simulink library "Common_Library"  (Simulink 8.1)
settings: Solver=ode45  StartTime=0.0  StopTime=10.0  RelTol=1e-3
values from neighbouring files (symbols this model uses):
  address_0x00 = MOVcr    [ROM.m]
  address_0x01 = 10    [ROM.m]
  address_0x02 = REG_A    [ROM.m]
  address_0x03 = MOVcr    [ROM.m]
  address_0x04 = 3    [ROM.m]
  address_0x05 = REG_B    [ROM.m]
  address_0x06 = ADDcr    [ROM.m]
  address_0x07 = 50    [ROM.m]
  address_0x08 = REG_B    [ROM.m]
  address_0x09 = ADDrr    [ROM.m]
  address_0x0A = REG_A    [ROM.m]
  address_0x0B = REG_B    [ROM.m]
  address_0x0C = 0    [ROM.m]
  address_0x0D = 0    [ROM.m]
  address_0x0E = 0    [ROM.m]
  address_0x0F = 177    [ROM.m]
libraries: Common_Library x115, Computer_Library x85, commutil2 x67, simulink_extras x1
(part 2 of 3)

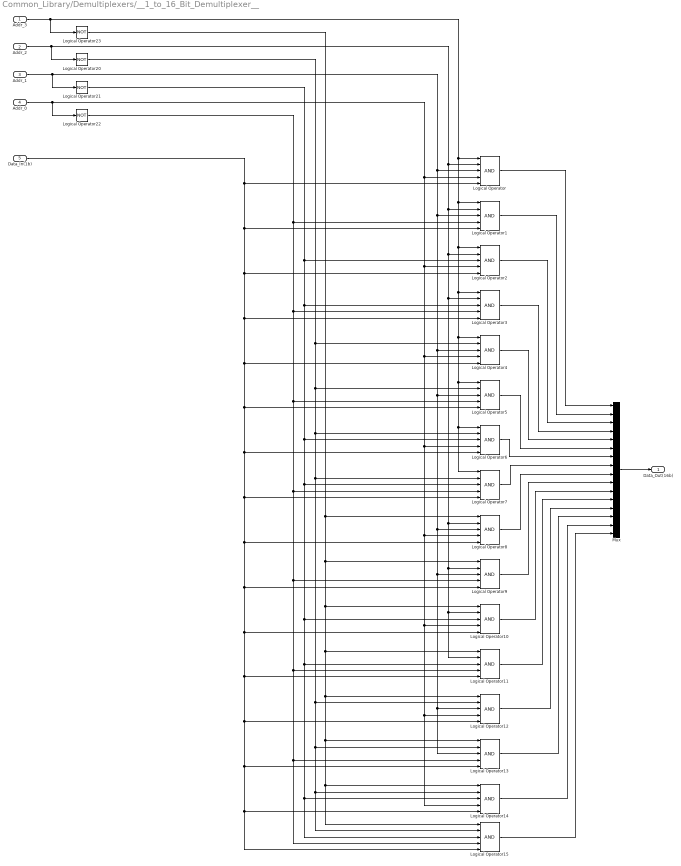
== system Common_Library/Demultiplexers/__1_to_16_Bit_Demultiplexer__ ==
  Addr_3 : Inport
  Addr_2 : Inport  Port=2
  Addr_1 : Inport  Port=3
  Addr_0 : Inport  Port=4
  Data_In(1b) : Inport  Port=5
  Logical Operator{,1..15} (16 alike) : Logic  Inputs=5  IconShape=distinctive  AllPortsSameDT=off  OutDataTypeStr=boolean
  Logical Operator{20..23} (4 alike) : Logic  Operator=NOT  Inputs=4  IconShape=distinctive  AllPortsSameDT=off  OutDataTypeStr=boolean
  Mux : Mux  Inputs=16
  Data_Out(16b) : Outport
  wires:
  Mux/1 -> Data_Out(16b)/1
  Logical Operator22/1 -> Logical Operator15/4, Logical Operator13/4, Logical Operator11/4, Logical Operator9/4, Logical Operator7/4, Logical Operator5/4, Logical Operator3/4, Logical Operator1/4
  Addr_0/1 -> Logical Operator14/4, Logical Operator12/4, Logical Operator10/4, Logical Operator8/4, Logical Operator6/4, Logical Operator4/4, Logical Operator2/4, Logical Operator/4, Logical Operator22/1
  Logical Operator21/1 -> Logical Operator15/3, Logical Operator14/3, Logical Operator11/3, Logical Operator10/3, Logical Operator7/3, Logical Operator6/3, Logical Operator3/3, Logical Operator2/3
  Addr_1/1 -> Logical Operator13/3, Logical Operator12/3, Logical Operator9/3, Logical Operator8/3, Logical Operator5/3, Logical Operator4/3, Logical Operator1/3, Logical Operator/3, Logical Operator21/1
  Logical Operator20/1 -> Logical Operator15/2, Logical Operator14/2, Logical Operator13/2, Logical Operator12/2, Logical Operator7/2, Logical Operator6/2, Logical Operator5/2, Logical Operator4/2
  Addr_2/1 -> Logical Operator11/2, Logical Operator10/2, Logical Operator9/2, Logical Operator8/2, Logical Operator3/2, Logical Operator2/2, Logical Operator1/2, Logical Operator/2, Logical Operator20/1
  Logical Operator23/1 -> Logical Operator15/1, Logical Operator14/1, Logical Operator13/1, Logical Operator12/1, Logical Operator11/1, Logical Operator10/1, Logical Operator9/1, Logical Operator8/1
  Addr_3/1 -> Logical Operator7/1, Logical Operator6/1, Logical Operator5/1, Logical Operator4/1, Logical Operator3/1, Logical Operator2/1, Logical Operator1/1, Logical Operator/1, Logical Operator23/1
  Data_In(1b)/1 -> Logical Operator/5, Logical Operator3/5, Logical Operator7/5, Logical Operator8/5, Logical Operator9/5, Logical Operator10/5, Logical Operator11/5, Logical Operator15/5, Logical Operator14/5, Logical Operator13/5, Logical Operator12/5, Logical Operator6/5, Logical Operator5/5, Logical Operator4/5, Logical Operator2/5, Logical Operator1/5
  Logical Operator15/1 -> Mux/16
  Logical Operator14/1 -> Mux/15
  Logical Operator13/1 -> Mux/14
  Logical Operator/1 -> Mux/1
  Logical Operator1/1 -> Mux/2
  Logical Operator2/1 -> Mux/3
  Logical Operator3/1 -> Mux/4
  Logical Operator4/1 -> Mux/5
  Logical Operator12/1 -> Mux/13
  Logical Operator11/1 -> Mux/12
  Logical Operator5/1 -> Mux/6
  Logical Operator10/1 -> Mux/11
  Logical Operator9/1 -> Mux/10
  Logical Operator6/1 -> Mux/7
  Logical Operator8/1 -> Mux/9
  Logical Operator7/1 -> Mux/8

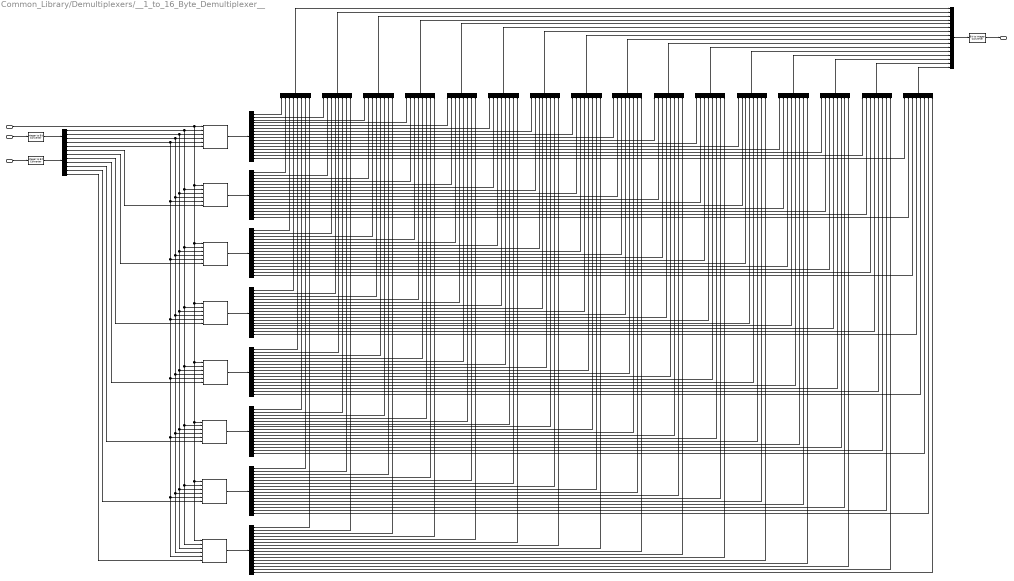
== system Common_Library/Demultiplexers/__1_to_16_Byte_Demultiplexer__ ==
  Enable : Inport
  Addr(4b) : Inport  Port=2
  Data_In(1B) : Inport  Port=3
  1_to_16_Bit_Demultiplexer(Bit_0) : Common_Library/Demultiplexers/1_to_16_Bit_Demultiplexer
  1_to_16_Bit_Demultiplexer(Bit_1) : Common_Library/Demultiplexers/1_to_16_Bit_Demultiplexer
  1_to_16_Bit_Demultiplexer(Bit_2) : Common_Library/Demultiplexers/1_to_16_Bit_Demultiplexer
  1_to_16_Bit_Demultiplexer(Bit_3) : Common_Library/Demultiplexers/1_to_16_Bit_Demultiplexer
  1_to_16_Bit_Demultiplexer(Bit_4) : Common_Library/Demultiplexers/1_to_16_Bit_Demultiplexer
  1_to_16_Bit_Demultiplexer(Bit_5) : Common_Library/Demultiplexers/1_to_16_Bit_Demultiplexer
  1_to_16_Bit_Demultiplexer(Bit_6) : Common_Library/Demultiplexers/1_to_16_Bit_Demultiplexer
  1_to_16_Bit_Demultiplexer(Bit_7) : Common_Library/Demultiplexers/1_to_16_Bit_Demultiplexer
  Bit to Integer Converter : commutil2/Bit to Integer Converter  nbits=8  bitOrder=MSB first  signedOutputValues=Unsigned  outDtype=uint8  outDtypeSigned=Inherit via internal rule
  Bit_{0..7} (8 alike) : Demux  Outputs=16
  Byte_{0..15} (16 alike) : Mux  Inputs=8
  Demux1 : Demux  Outputs=8
  Demux17 : Demux
  Integer to Bit Converter5 : commutil2/Integer to Bit Converter  nbits=4  signedInputValues=Unsigned  bitOrder=MSB first  outDtype=int8
  Integer to Bit Converter7 : commutil2/Integer to Bit Converter  nbits=8  signedInputValues=Unsigned  bitOrder=MSB first  outDtype=boolean
  Mux1 : Mux  Inputs=16
  Data_Out(16B) : Outport
  wires:
  Bit to Integer Converter/1 -> Data_Out(16B)/1
  Mux1/1 -> Bit to Integer Converter/1
  Addr(4b)/1 -> Integer to Bit Converter5/1
  Integer to Bit Converter5/1 -> Demux17/1
  Enable/1 -> 1_to_16_Bit_Demultiplexer(Bit_0)/1, 1_to_16_Bit_Demultiplexer(Bit_1)/1, 1_to_16_Bit_Demultiplexer(Bit_2)/1, 1_to_16_Bit_Demultiplexer(Bit_3)/1, 1_to_16_Bit_Demultiplexer(Bit_4)/1, 1_to_16_Bit_Demultiplexer(Bit_5)/1, 1_to_16_Bit_Demultiplexer(Bit_6)/1, 1_to_16_Bit_Demultiplexer(Bit_7)/1
  Demux1/4 -> 1_to_16_Bit_Demultiplexer(Bit_4)/6
  Demux1/5 -> 1_to_16_Bit_Demultiplexer(Bit_3)/6
  Demux1/6 -> 1_to_16_Bit_Demultiplexer(Bit_2)/6
  Demux1/7 -> 1_to_16_Bit_Demultiplexer(Bit_1)/6
  Demux1/8 -> 1_to_16_Bit_Demultiplexer(Bit_0)/6
  Demux1/3 -> 1_to_16_Bit_Demultiplexer(Bit_5)/6
  Demux1/2 -> 1_to_16_Bit_Demultiplexer(Bit_6)/6
  Demux1/1 -> 1_to_16_Bit_Demultiplexer(Bit_7)/6
  Byte_15/1 -> Mux1/1
  Byte_14/1 -> Mux1/2
  Byte_13/1 -> Mux1/3
  Byte_12/1 -> Mux1/4
  Byte_11/1 -> Mux1/5
  Byte_10/1 -> Mux1/6
  Byte_9/1 -> Mux1/7
  Byte_8/1 -> Mux1/8
  Byte_7/1 -> Mux1/9
  Byte_6/1 -> Mux1/10
  Byte_5/1 -> Mux1/11
  Byte_4/1 -> Mux1/12
  Byte_3/1 -> Mux1/13
  Byte_2/1 -> Mux1/14
  Byte_1/1 -> Mux1/15
  Byte_0/1 -> Mux1/16
  Bit_0/16 -> Byte_0/8
  Bit_0/15 -> Byte_1/8
  Bit_0/14 -> Byte_2/8
  Bit_0/13 -> Byte_3/8
  Bit_0/12 -> Byte_4/8
  Bit_0/11 -> Byte_5/8
  Bit_0/10 -> Byte_6/8
  Bit_0/9 -> Byte_7/8
  Bit_0/8 -> Byte_8/8
  Bit_0/7 -> Byte_9/8
  Bit_0/6 -> Byte_10/8
  Bit_0/5 -> Byte_11/8
  Bit_0/4 -> Byte_12/8
  Bit_0/3 -> Byte_13/8
  Bit_0/2 -> Byte_14/8
  Bit_0/1 -> Byte_15/8
  Bit_1/16 -> Byte_0/7
  Bit_1/15 -> Byte_1/7
  Bit_1/14 -> Byte_2/7
  Bit_1/13 -> Byte_3/7
  Bit_1/12 -> Byte_4/7
  Bit_1/11 -> Byte_5/7
  Bit_1/10 -> Byte_6/7
  Bit_1/9 -> Byte_7/7
  Bit_1/8 -> Byte_8/7
  Bit_1/7 -> Byte_9/7
  Bit_1/6 -> Byte_10/7
  Bit_1/5 -> Byte_11/7
  Bit_1/4 -> Byte_12/7
  Bit_1/3 -> Byte_13/7
  Bit_1/2 -> Byte_14/7
  Bit_1/1 -> Byte_15/7
  Bit_2/16 -> Byte_0/6
  Bit_2/15 -> Byte_1/6
  Bit_2/14 -> Byte_2/6
  Bit_2/13 -> Byte_3/6
  Bit_2/12 -> Byte_4/6
  Bit_2/11 -> Byte_5/6
  Bit_2/10 -> Byte_6/6
  Bit_2/9 -> Byte_7/6
  Bit_2/8 -> Byte_8/6
  Bit_2/7 -> Byte_9/6
  Bit_2/6 -> Byte_10/6
  Bit_2/5 -> Byte_11/6
  Bit_2/4 -> Byte_12/6
  Bit_2/3 -> Byte_13/6
  Bit_2/2 -> Byte_14/6
  Bit_2/1 -> Byte_15/6
  Bit_3/16 -> Byte_0/5
  Bit_3/15 -> Byte_1/5
  Bit_3/14 -> Byte_2/5
  Bit_3/13 -> Byte_3/5
  Bit_3/12 -> Byte_4/5
  Bit_3/11 -> Byte_5/5
  Bit_3/10 -> Byte_6/5
  Bit_3/9 -> Byte_7/5
  Bit_3/8 -> Byte_8/5
  Bit_3/7 -> Byte_9/5
  Bit_3/6 -> Byte_10/5
  Bit_3/5 -> Byte_11/5
  Bit_3/4 -> Byte_12/5
  Bit_3/3 -> Byte_13/5
  Bit_3/2 -> Byte_14/5
  Bit_3/1 -> Byte_15/5
  Bit_4/16 -> Byte_0/4
  Bit_4/15 -> Byte_1/4
  Bit_4/14 -> Byte_2/4
  Bit_4/13 -> Byte_3/4
  Bit_4/12 -> Byte_4/4
  Bit_4/11 -> Byte_5/4
  Bit_4/10 -> Byte_6/4
  Bit_4/9 -> Byte_7/4
  Bit_4/8 -> Byte_8/4
  Bit_4/7 -> Byte_9/4
  Bit_4/6 -> Byte_10/4
  Bit_4/5 -> Byte_11/4
  Bit_4/4 -> Byte_12/4
  Bit_4/3 -> Byte_13/4
  Bit_4/2 -> Byte_14/4
  Bit_4/1 -> Byte_15/4
  Bit_5/16 -> Byte_0/3
  Bit_5/15 -> Byte_1/3
  Bit_5/14 -> Byte_2/3
  Bit_5/13 -> Byte_3/3
  Bit_5/12 -> Byte_4/3
  Bit_5/11 -> Byte_5/3
  Bit_5/10 -> Byte_6/3
  Bit_5/9 -> Byte_7/3
  Bit_5/8 -> Byte_8/3
  Bit_5/7 -> Byte_9/3
  Bit_5/6 -> Byte_10/3
  Bit_5/5 -> Byte_11/3
  Bit_5/4 -> Byte_12/3
  Bit_5/3 -> Byte_13/3
  Bit_5/2 -> Byte_14/3
  Bit_5/1 -> Byte_15/3
  Bit_6/16 -> Byte_0/2
  Bit_6/15 -> Byte_1/2
  Bit_6/14 -> Byte_2/2
  Bit_6/13 -> Byte_3/2
  Bit_6/12 -> Byte_4/2
  Bit_6/11 -> Byte_5/2
  Bit_6/10 -> Byte_6/2
  Bit_6/9 -> Byte_7/2
  Bit_6/8 -> Byte_8/2
  Bit_6/7 -> Byte_9/2
  Bit_6/6 -> Byte_10/2
  Bit_6/5 -> Byte_11/2
  Bit_6/4 -> Byte_12/2
  Bit_6/3 -> Byte_13/2
  Bit_6/2 -> Byte_14/2
  Bit_6/1 -> Byte_15/2
  Bit_7/16 -> Byte_0/1
  Bit_7/15 -> Byte_1/1
  Bit_7/14 -> Byte_2/1
  Bit_7/13 -> Byte_3/1
  Bit_7/12 -> Byte_4/1
  Bit_7/11 -> Byte_5/1
  Bit_7/10 -> Byte_6/1
  Bit_7/9 -> Byte_7/1
  Bit_7/8 -> Byte_8/1
  Bit_7/7 -> Byte_9/1
  Bit_7/6 -> Byte_10/1
  Bit_7/5 -> Byte_11/1
  Bit_7/4 -> Byte_12/1
  Bit_7/3 -> Byte_13/1
  Bit_7/2 -> Byte_14/1
  Bit_7/1 -> Byte_15/1
  1_to_16_Bit_Demultiplexer(Bit_0)/1 -> Bit_0/1
  1_to_16_Bit_Demultiplexer(Bit_1)/1 -> Bit_1/1
  1_to_16_Bit_Demultiplexer(Bit_2)/1 -> Bit_2/1
  1_to_16_Bit_Demultiplexer(Bit_3)/1 -> Bit_3/1
  1_to_16_Bit_Demultiplexer(Bit_4)/1 -> Bit_4/1
  1_to_16_Bit_Demultiplexer(Bit_5)/1 -> Bit_5/1
  1_to_16_Bit_Demultiplexer(Bit_6)/1 -> Bit_6/1
  1_to_16_Bit_Demultiplexer(Bit_7)/1 -> Bit_7/1
  Integer to Bit Converter7/1 -> Demux1/1
  Data_In(1B)/1 -> Integer to Bit Converter7/1
  Demux17/4 -> 1_to_16_Bit_Demultiplexer(Bit_7)/5, 1_to_16_Bit_Demultiplexer(Bit_0)/5, 1_to_16_Bit_Demultiplexer(Bit_1)/5, 1_to_16_Bit_Demultiplexer(Bit_2)/5, 1_to_16_Bit_Demultiplexer(Bit_3)/5, 1_to_16_Bit_Demultiplexer(Bit_4)/5, 1_to_16_Bit_Demultiplexer(Bit_5)/5, 1_to_16_Bit_Demultiplexer(Bit_6)/5
  Demux17/3 -> 1_to_16_Bit_Demultiplexer(Bit_7)/4, 1_to_16_Bit_Demultiplexer(Bit_0)/4, 1_to_16_Bit_Demultiplexer(Bit_1)/4, 1_to_16_Bit_Demultiplexer(Bit_2)/4, 1_to_16_Bit_Demultiplexer(Bit_3)/4, 1_to_16_Bit_Demultiplexer(Bit_4)/4, 1_to_16_Bit_Demultiplexer(Bit_5)/4, 1_to_16_Bit_Demultiplexer(Bit_6)/4
  Demux17/2 -> 1_to_16_Bit_Demultiplexer(Bit_7)/3, 1_to_16_Bit_Demultiplexer(Bit_1)/3, 1_to_16_Bit_Demultiplexer(Bit_0)/3, 1_to_16_Bit_Demultiplexer(Bit_2)/3, 1_to_16_Bit_Demultiplexer(Bit_3)/3, 1_to_16_Bit_Demultiplexer(Bit_4)/3, 1_to_16_Bit_Demultiplexer(Bit_5)/3, 1_to_16_Bit_Demultiplexer(Bit_6)/3
  Demux17/1 -> 1_to_16_Bit_Demultiplexer(Bit_7)/2, 1_to_16_Bit_Demultiplexer(Bit_0)/2, 1_to_16_Bit_Demultiplexer(Bit_1)/2, 1_to_16_Bit_Demultiplexer(Bit_2)/2, 1_to_16_Bit_Demultiplexer(Bit_3)/2, 1_to_16_Bit_Demultiplexer(Bit_4)/2, 1_to_16_Bit_Demultiplexer(Bit_5)/2, 1_to_16_Bit_Demultiplexer(Bit_6)/2

== system Common_Library/Demultiplexers/__1_to_256_Bit_Demultiplexer__ ==
  Address(8b) : Inport
  Data_In(1b) : Inport  Port=2
  1_to_16_Bit_Demultiplexer{,1..16} (17 alike) : Computer_Library/Demultiplexers/1_to_16_Bit_Demultiplexer
  Constant : Constant
  Demux1 : Demux  Outputs=16
  Demux17 : Demux  Outputs=8
  Mux : Mux  Inputs=16
  Data_Out(256b) : Outport  OutDataTypeStr=boolean
  wires:
  Mux/1 -> Data_Out(256b)/1
  Constant/1 -> 1_to_16_Bit_Demultiplexer16/1
  Demux17/4 -> 1_to_16_Bit_Demultiplexer16/5
  Demux17/3 -> 1_to_16_Bit_Demultiplexer16/4
  Demux17/2 -> 1_to_16_Bit_Demultiplexer16/3
  Demux17/1 -> 1_to_16_Bit_Demultiplexer16/2
  Demux1/16 -> 1_to_16_Bit_Demultiplexer15/1
  Demux1/15 -> 1_to_16_Bit_Demultiplexer14/1
  Demux1/14 -> 1_to_16_Bit_Demultiplexer13/1
  Demux1/13 -> 1_to_16_Bit_Demultiplexer12/1
  Demux1/12 -> 1_to_16_Bit_Demultiplexer11/1
  Demux1/11 -> 1_to_16_Bit_Demultiplexer10/1
  Demux1/10 -> 1_to_16_Bit_Demultiplexer9/1
  Demux1/9 -> 1_to_16_Bit_Demultiplexer8/1
  Demux1/8 -> 1_to_16_Bit_Demultiplexer7/1
  Demux1/7 -> 1_to_16_Bit_Demultiplexer6/1
  Demux1/6 -> 1_to_16_Bit_Demultiplexer5/1
  Demux1/5 -> 1_to_16_Bit_Demultiplexer4/1
  Demux1/4 -> 1_to_16_Bit_Demultiplexer3/1
  Demux1/3 -> 1_to_16_Bit_Demultiplexer2/1
  Demux1/2 -> 1_to_16_Bit_Demultiplexer1/1
  Demux1/1 -> 1_to_16_Bit_Demultiplexer/1
  1_to_16_Bit_Demultiplexer16/1 -> Demux1/1
  Data_In(1b)/1 -> 1_to_16_Bit_Demultiplexer16/6, 1_to_16_Bit_Demultiplexer/6, 1_to_16_Bit_Demultiplexer2/6, 1_to_16_Bit_Demultiplexer3/6, 1_to_16_Bit_Demultiplexer4/6, 1_to_16_Bit_Demultiplexer5/6, 1_to_16_Bit_Demultiplexer6/6, 1_to_16_Bit_Demultiplexer7/6, 1_to_16_Bit_Demultiplexer8/6, 1_to_16_Bit_Demultiplexer9/6, 1_to_16_Bit_Demultiplexer10/6, 1_to_16_Bit_Demultiplexer11/6, 1_to_16_Bit_Demultiplexer12/6, 1_to_16_Bit_Demultiplexer13/6, 1_to_16_Bit_Demultiplexer14/6, 1_to_16_Bit_Demultiplexer15/6, 1_to_16_Bit_Demultiplexer1/6
  1_to_16_Bit_Demultiplexer/1 -> Mux/1
  1_to_16_Bit_Demultiplexer1/1 -> Mux/2
  1_to_16_Bit_Demultiplexer2/1 -> Mux/3
  1_to_16_Bit_Demultiplexer3/1 -> Mux/4
  1_to_16_Bit_Demultiplexer15/1 -> Mux/16
  1_to_16_Bit_Demultiplexer14/1 -> Mux/15
  1_to_16_Bit_Demultiplexer13/1 -> Mux/14
  1_to_16_Bit_Demultiplexer12/1 -> Mux/13
  1_to_16_Bit_Demultiplexer11/1 -> Mux/12
  1_to_16_Bit_Demultiplexer10/1 -> Mux/11
  1_to_16_Bit_Demultiplexer9/1 -> Mux/10
  1_to_16_Bit_Demultiplexer8/1 -> Mux/9
  1_to_16_Bit_Demultiplexer7/1 -> Mux/8
  1_to_16_Bit_Demultiplexer6/1 -> Mux/7
  1_to_16_Bit_Demultiplexer5/1 -> Mux/6
  1_to_16_Bit_Demultiplexer4/1 -> Mux/5
  Demux17/5 -> 1_to_16_Bit_Demultiplexer/2, 1_to_16_Bit_Demultiplexer7/2, 1_to_16_Bit_Demultiplexer9/2, 1_to_16_Bit_Demultiplexer10/2, 1_to_16_Bit_Demultiplexer14/2, 1_to_16_Bit_Demultiplexer15/2, 1_to_16_Bit_Demultiplexer13/2, 1_to_16_Bit_Demultiplexer12/2, 1_to_16_Bit_Demultiplexer11/2, 1_to_16_Bit_Demultiplexer8/2, 1_to_16_Bit_Demultiplexer6/2, 1_to_16_Bit_Demultiplexer5/2, 1_to_16_Bit_Demultiplexer4/2, 1_to_16_Bit_Demultiplexer3/2, 1_to_16_Bit_Demultiplexer2/2, 1_to_16_Bit_Demultiplexer1/2
  Demux17/6 -> 1_to_16_Bit_Demultiplexer/3, 1_to_16_Bit_Demultiplexer3/3, 1_to_16_Bit_Demultiplexer4/3, 1_to_16_Bit_Demultiplexer7/3, 1_to_16_Bit_Demultiplexer8/3, 1_to_16_Bit_Demultiplexer9/3, 1_to_16_Bit_Demultiplexer10/3, 1_to_16_Bit_Demultiplexer12/3, 1_to_16_Bit_Demultiplexer14/3, 1_to_16_Bit_Demultiplexer15/3, 1_to_16_Bit_Demultiplexer13/3, 1_to_16_Bit_Demultiplexer11/3, 1_to_16_Bit_Demultiplexer6/3, 1_to_16_Bit_Demultiplexer5/3, 1_to_16_Bit_Demultiplexer2/3, 1_to_16_Bit_Demultiplexer1/3
  Demux17/7 -> 1_to_16_Bit_Demultiplexer/4, 1_to_16_Bit_Demultiplexer2/4, 1_to_16_Bit_Demultiplexer3/4, 1_to_16_Bit_Demultiplexer4/4, 1_to_16_Bit_Demultiplexer7/4, 1_to_16_Bit_Demultiplexer8/4, 1_to_16_Bit_Demultiplexer9/4, 1_to_16_Bit_Demultiplexer10/4, 1_to_16_Bit_Demultiplexer12/4, 1_to_16_Bit_Demultiplexer14/4, 1_to_16_Bit_Demultiplexer15/4, 1_to_16_Bit_Demultiplexer13/4, 1_to_16_Bit_Demultiplexer11/4, 1_to_16_Bit_Demultiplexer6/4, 1_to_16_Bit_Demultiplexer5/4, 1_to_16_Bit_Demultiplexer1/4
  Demux17/8 -> 1_to_16_Bit_Demultiplexer/5, 1_to_16_Bit_Demultiplexer1/5, 1_to_16_Bit_Demultiplexer2/5, 1_to_16_Bit_Demultiplexer3/5, 1_to_16_Bit_Demultiplexer4/5, 1_to_16_Bit_Demultiplexer5/5, 1_to_16_Bit_Demultiplexer7/5, 1_to_16_Bit_Demultiplexer8/5, 1_to_16_Bit_Demultiplexer9/5, 1_to_16_Bit_Demultiplexer10/5, 1_to_16_Bit_Demultiplexer12/5, 1_to_16_Bit_Demultiplexer14/5, 1_to_16_Bit_Demultiplexer15/5, 1_to_16_Bit_Demultiplexer13/5, 1_to_16_Bit_Demultiplexer11/5, 1_to_16_Bit_Demultiplexer6/5
  Address(8b)/1 -> Demux17/1

== system Common_Library/Demultiplexers/__1_to_256_Byte_Demultiplexer__ ==
  Address(8b) : Inport
  Data_In(1B) : Inport  Port=2
  1_to_16_Bit_Demultiplexer16 : Computer_Library/Demultiplexers/1_to_16_Bit_Demultiplexer
  1_to_16_Byte_Demultiplexer{,1..15} (16 alike) : Computer_Library/Demultiplexers/1_to_16_Byte_Demultiplexer
  Bit to Integer Converter : commutil2/Bit to Integer Converter  nbits=4  bitOrder=MSB first  signedOutputValues=Unsigned  outDtype=uint8  outDtypeSigned=Inherit via internal rule
  Constant : Constant
  Demux1 : Demux  Outputs=16
  Demux17 : Demux  Outputs=8
  Integer to Bit Converter7 : commutil2/Integer to Bit Converter  nbits=8  signedInputValues=Unsigned  bitOrder=MSB first  outDtype=boolean
  Mux : Mux  Inputs=16
  Mux1 : Mux
  Data_Out(256B) : Outport  OutDataTypeStr=uint8
  wires:
  Mux1/1 -> Bit to Integer Converter/1
  Address(8b)/1 -> Integer to Bit Converter7/1
  Integer to Bit Converter7/1 -> Demux17/1
  Bit to Integer Converter/1 -> 1_to_16_Byte_Demultiplexer2/2, 1_to_16_Byte_Demultiplexer3/2, 1_to_16_Byte_Demultiplexer4/2, 1_to_16_Byte_Demultiplexer15/2, 1_to_16_Byte_Demultiplexer14/2, 1_to_16_Byte_Demultiplexer13/2, 1_to_16_Byte_Demultiplexer12/2, 1_to_16_Byte_Demultiplexer11/2, 1_to_16_Byte_Demultiplexer10/2, 1_to_16_Byte_Demultiplexer9/2, 1_to_16_Byte_Demultiplexer8/2, 1_to_16_Byte_Demultiplexer7/2, 1_to_16_Byte_Demultiplexer6/2, 1_to_16_Byte_Demultiplexer5/2, 1_to_16_Byte_Demultiplexer1/2, 1_to_16_Byte_Demultiplexer/2
  Demux17/8 -> Mux1/4
  Demux17/7 -> Mux1/3
  Demux17/6 -> Mux1/2
  Demux17/5 -> Mux1/1
  Demux17/3 -> 1_to_16_Bit_Demultiplexer16/4
  Demux17/4 -> 1_to_16_Bit_Demultiplexer16/5
  Demux17/2 -> 1_to_16_Bit_Demultiplexer16/3
  Demux17/1 -> 1_to_16_Bit_Demultiplexer16/2
  Mux/1 -> Data_Out(256B)/1
  Constant/1 -> 1_to_16_Bit_Demultiplexer16/6, 1_to_16_Bit_Demultiplexer16/1
  Demux1/16 -> 1_to_16_Byte_Demultiplexer15/1
  Demux1/15 -> 1_to_16_Byte_Demultiplexer14/1
  Demux1/14 -> 1_to_16_Byte_Demultiplexer13/1
  Demux1/13 -> 1_to_16_Byte_Demultiplexer12/1
  Demux1/12 -> 1_to_16_Byte_Demultiplexer11/1
  Demux1/11 -> 1_to_16_Byte_Demultiplexer10/1
  Demux1/10 -> 1_to_16_Byte_Demultiplexer9/1
  Demux1/9 -> 1_to_16_Byte_Demultiplexer8/1
  Demux1/8 -> 1_to_16_Byte_Demultiplexer7/1
  Demux1/7 -> 1_to_16_Byte_Demultiplexer6/1
  Demux1/6 -> 1_to_16_Byte_Demultiplexer5/1
  Demux1/5 -> 1_to_16_Byte_Demultiplexer4/1
  Demux1/4 -> 1_to_16_Byte_Demultiplexer3/1
  Demux1/3 -> 1_to_16_Byte_Demultiplexer2/1
  Demux1/2 -> 1_to_16_Byte_Demultiplexer1/1
  Demux1/1 -> 1_to_16_Byte_Demultiplexer/1
  1_to_16_Bit_Demultiplexer16/1 -> Demux1/1
  Data_In(1B)/1 -> 1_to_16_Byte_Demultiplexer/3, 1_to_16_Byte_Demultiplexer1/3, 1_to_16_Byte_Demultiplexer2/3, 1_to_16_Byte_Demultiplexer3/3, 1_to_16_Byte_Demultiplexer4/3, 1_to_16_Byte_Demultiplexer5/3, 1_to_16_Byte_Demultiplexer6/3, 1_to_16_Byte_Demultiplexer7/3, 1_to_16_Byte_Demultiplexer8/3, 1_to_16_Byte_Demultiplexer9/3, 1_to_16_Byte_Demultiplexer10/3, 1_to_16_Byte_Demultiplexer11/3, 1_to_16_Byte_Demultiplexer12/3, 1_to_16_Byte_Demultiplexer13/3, 1_to_16_Byte_Demultiplexer14/3, 1_to_16_Byte_Demultiplexer15/3
  1_to_16_Byte_Demultiplexer/1 -> Mux/1
  1_to_16_Byte_Demultiplexer1/1 -> Mux/2
  1_to_16_Byte_Demultiplexer2/1 -> Mux/3
  1_to_16_Byte_Demultiplexer3/1 -> Mux/4
  1_to_16_Byte_Demultiplexer15/1 -> Mux/16
  1_to_16_Byte_Demultiplexer14/1 -> Mux/15
  1_to_16_Byte_Demultiplexer13/1 -> Mux/14
  1_to_16_Byte_Demultiplexer12/1 -> Mux/13
  1_to_16_Byte_Demultiplexer11/1 -> Mux/12
  1_to_16_Byte_Demultiplexer10/1 -> Mux/11
  1_to_16_Byte_Demultiplexer9/1 -> Mux/10
  1_to_16_Byte_Demultiplexer8/1 -> Mux/9
  1_to_16_Byte_Demultiplexer7/1 -> Mux/8
  1_to_16_Byte_Demultiplexer6/1 -> Mux/7
  1_to_16_Byte_Demultiplexer5/1 -> Mux/6
  1_to_16_Byte_Demultiplexer4/1 -> Mux/5

== system Common_Library/Encoders/4_to_2_Encoder ==
  Select_3(1b) : Inport
  "Select_2(1b) " : Inport  Port=2
  Select_1(1b) : Inport  Port=3
  Select_0(1b) : Inport  Port=4
  Logical Operator : Logic  Operator=OR  IconShape=distinctive  AllPortsSameDT=off  OutDataTypeStr=boolean
  Logical Operator1 : Logic  Operator=OR  IconShape=distinctive  AllPortsSameDT=off  OutDataTypeStr=boolean
  Terminator : Terminator
  Address_Out_1(1b) : Outport
  Address_Out_0(1b) : Outport  Port=2
  wires:
  Select_3(1b)/1 -> Logical Operator1/1, Logical Operator/1
  Select_0(1b)/1 -> Terminator/1
  Select_1(1b)/1 -> Logical Operator1/2
  "Select_2(1b) "/1 -> Logical Operator/2
  Logical Operator1/1 -> Address_Out_0(1b)/1
  Logical Operator/1 -> Address_Out_1(1b)/1

== system Common_Library/Encoders/__16_to_4_Encoder__ ==
  In_0 : Inport
  "In_1 " : Inport  Port=2
  In_2 : Inport  Port=3
  In_3 : Inport  Port=4
  In_4 : Inport  Port=5
  In_5 : Inport  Port=6
  In_6 : Inport  Port=7
  In_7 : Inport  Port=8
  In_8 : Inport  Port=9
  In_9 : Inport  Port=10
  In_10 : Inport  Port=11
  In_11 : Inport  Port=12
  In_12 : Inport  Port=13
  In_13 : Inport  Port=14
  In_14 : Inport  Port=15
  In_15 : Inport  Port=16
  Logical Operator{,1..3} (4 alike) : Logic  Operator=OR  Inputs=8  IconShape=distinctive  AllPortsSameDT=off  OutDataTypeStr=boolean
  Terminator : Terminator
  Out_0 : Outport
  Out_1 : Outport  Port=2
  Out_2 : Outport  Port=3
  Out_3 : Outport  Port=4
  wires:
  In_0/1 -> Terminator/1
  In_15/1 -> Logical Operator/8, Logical Operator1/8, Logical Operator2/8, Logical Operator3/8
  In_14/1 -> Logical Operator1/7, Logical Operator2/7, Logical Operator3/7
  In_13/1 -> Logical Operator/7, Logical Operator2/6, Logical Operator3/6
  In_12/1 -> Logical Operator2/5, Logical Operator3/5
  In_11/1 -> Logical Operator/6, Logical Operator1/6, Logical Operator3/4
  In_10/1 -> Logical Operator1/5, Logical Operator3/3
  In_9/1 -> Logical Operator/5, Logical Operator3/2
  In_8/1 -> Logical Operator3/1
  In_7/1 -> Logical Operator/4, Logical Operator1/4, Logical Operator2/4
  In_6/1 -> Logical Operator1/3, Logical Operator2/3
  In_5/1 -> Logical Operator/3, Logical Operator2/2
  In_4/1 -> Logical Operator2/1
  In_3/1 -> Logical Operator/2, Logical Operator1/2
  In_2/1 -> Logical Operator1/1
  "In_1 "/1 -> Logical Operator/1
  Logical Operator3/1 -> Out_3/1
  Logical Operator2/1 -> Out_2/1
  Logical Operator1/1 -> Out_1/1
  Logical Operator/1 -> Out_0/1

== system Common_Library/Encoders/__8_to_3_Encoder__ ==
  In_0 : Inport
  "In_1 " : Inport  Port=2
  In_2 : Inport  Port=3
  In_3 : Inport  Port=4
  In_4 : Inport  Port=5
  In_5 : Inport  Port=6
  In_6 : Inport  Port=7
  In_7 : Inport  Port=8
  Logical Operator : Logic  Operator=OR  Inputs=4  IconShape=distinctive  AllPortsSameDT=off  OutDataTypeStr=boolean
  Logical Operator1 : Logic  Operator=OR  Inputs=4  IconShape=distinctive  AllPortsSameDT=off  OutDataTypeStr=boolean
  Logical Operator2 : Logic  Operator=OR  Inputs=4  IconShape=distinctive  AllPortsSameDT=off  OutDataTypeStr=boolean
  Terminator : Terminator
  Out_0 : Outport
  Out_1 : Outport  Port=2
  Out_2 : Outport  Port=3
  wires:
  In_0/1 -> Terminator/1
  In_7/1 -> Logical Operator/4, Logical Operator1/4, Logical Operator2/4
  In_6/1 -> Logical Operator1/3, Logical Operator2/3
  In_5/1 -> Logical Operator/3, Logical Operator2/2
  In_4/1 -> Logical Operator2/1
  In_3/1 -> Logical Operator/2, Logical Operator1/2
  In_2/1 -> Logical Operator1/1
  "In_1 "/1 -> Logical Operator/1
  Logical Operator2/1 -> Out_2/1
  Logical Operator1/1 -> Out_1/1
  Logical Operator/1 -> Out_0/1

== system Common_Library/Memory_Blocks/16B_RAM_Memory ==
  Addr_3(1b) : Inport
  Addr_2(1b) : Inport  Port=2
  Addr_1(1b) : Inport  Port=3
  Addr_0(1b) : Inport  Port=4
  Write(1b) : Inport  Port=5
  Data_In(1B) : Inport  Port=6
  CLK : Inport  Port=7  OutDataTypeStr=double
  16_to_1_Byte_Multiplexer : Common_Library/Multiplexers/16_to_1_Byte_Multiplexer
  4_to_16_Decoder : Common_Library/Decoders/4_to_16_Decoder
  Byte{0..15} (16 alike) : Common_Library/Memory_Blocks/Byte
  Data_Out(1B) : Outport
  wires:
  16_to_1_Byte_Multiplexer/1 -> Data_Out(1B)/1
  Byte0/1 -> 16_to_1_Byte_Multiplexer/20
  Byte1/1 -> 16_to_1_Byte_Multiplexer/19
  Byte2/1 -> 16_to_1_Byte_Multiplexer/18
  Byte3/1 -> 16_to_1_Byte_Multiplexer/17
  Byte4/1 -> 16_to_1_Byte_Multiplexer/16
  Byte5/1 -> 16_to_1_Byte_Multiplexer/15
  Byte6/1 -> 16_to_1_Byte_Multiplexer/14
  Byte7/1 -> 16_to_1_Byte_Multiplexer/13
  Byte8/1 -> 16_to_1_Byte_Multiplexer/12
  Byte9/1 -> 16_to_1_Byte_Multiplexer/11
  Byte10/1 -> 16_to_1_Byte_Multiplexer/10
  Byte11/1 -> 16_to_1_Byte_Multiplexer/9
  Byte12/1 -> 16_to_1_Byte_Multiplexer/8
  Byte13/1 -> 16_to_1_Byte_Multiplexer/7
  Byte14/1 -> 16_to_1_Byte_Multiplexer/6
  Byte15/1 -> 16_to_1_Byte_Multiplexer/5
  4_to_16_Decoder/16 -> Byte0/1
  4_to_16_Decoder/15 -> Byte1/1
  4_to_16_Decoder/14 -> Byte2/1
  4_to_16_Decoder/13 -> Byte3/1
  4_to_16_Decoder/12 -> Byte4/1
  4_to_16_Decoder/11 -> Byte5/1
  4_to_16_Decoder/10 -> Byte6/1
  4_to_16_Decoder/9 -> Byte7/1
  4_to_16_Decoder/8 -> Byte8/1
  4_to_16_Decoder/7 -> Byte9/1
  4_to_16_Decoder/6 -> Byte10/1
  4_to_16_Decoder/5 -> Byte11/1
  4_to_16_Decoder/4 -> Byte12/1
  4_to_16_Decoder/3 -> Byte13/1
  4_to_16_Decoder/2 -> Byte14/1
  Addr_3(1b)/1 -> 16_to_1_Byte_Multiplexer/1, 4_to_16_Decoder/1
  4_to_16_Decoder/1 -> Byte15/1
  Write(1b)/1 -> Byte15/2, Byte14/2, Byte13/2, Byte12/2, Byte11/2, Byte10/2, Byte9/2, Byte8/2, Byte7/2, Byte6/2, Byte5/2, Byte4/2, Byte3/2, Byte2/2, Byte1/2, Byte0/2
  Data_In(1B)/1 -> Byte15/3, Byte14/3, Byte13/3, Byte12/3, Byte11/3, Byte10/3, Byte9/3, Byte8/3, Byte7/3, Byte6/3, Byte5/3, Byte4/3, Byte3/3, Byte2/3, Byte1/3, Byte0/3
  CLK/1 -> Byte15/4, Byte14/4, Byte13/4, Byte12/4, Byte11/4, Byte10/4, Byte9/4, Byte8/4, Byte7/4, Byte6/4, Byte5/4, Byte4/4, Byte3/4, Byte2/4, Byte1/4, Byte0/4
  Addr_2(1b)/1 -> 16_to_1_Byte_Multiplexer/2, 4_to_16_Decoder/2
  Addr_1(1b)/1 -> 16_to_1_Byte_Multiplexer/3, 4_to_16_Decoder/3
  Addr_0(1b)/1 -> 16_to_1_Byte_Multiplexer/4, 4_to_16_Decoder/4

== system Common_Library/Memory_Blocks/16B_ROM_Memory ==
  Addr_3(1b) : Inport
  Addr_2(1b) : Inport  Port=2
  Addr_1(1b) : Inport  Port=3
  Addr_0(1b) : Inport  Port=4
  16_to_1_Byte_Multiplexer : Common_Library/Multiplexers/16_to_1_Byte_Multiplexer
  Byte_00 : Constant  Value=address_0x00  OutDataTypeStr=uint8
  Byte_01 : Constant  Value=address_0x01  OutDataTypeStr=uint8
  Byte_02 : Constant  Value=address_0x02  OutDataTypeStr=uint8
  Byte_03 : Constant  Value=address_0x03  OutDataTypeStr=uint8
  Byte_04 : Constant  Value=address_0x04  OutDataTypeStr=uint8
  Byte_05 : Constant  Value=address_0x05  OutDataTypeStr=uint8
  Byte_06 : Constant  Value=address_0x06  OutDataTypeStr=uint8
  Byte_07 : Constant  Value=address_0x07  OutDataTypeStr=uint8
  Byte_08 : Constant  Value=address_0x08  OutDataTypeStr=uint8
  Byte_09 : Constant  Value=address_0x09  OutDataTypeStr=uint8
  Byte_10 : Constant  Value=address_0x0A  OutDataTypeStr=uint8
  Byte_11 : Constant  Value=address_0x0B  OutDataTypeStr=uint8
  Byte_12 : Constant  Value=address_0x0C  OutDataTypeStr=uint8
  Byte_13 : Constant  Value=address_0x0D  OutDataTypeStr=uint8
  Byte_14 : Constant  Value=address_0x0E  OutDataTypeStr=uint8
  Byte_15 : Constant  Value=address_0x0F  OutDataTypeStr=uint8
  Data_Out(1B) : Outport
  wires:
  16_to_1_Byte_Multiplexer/1 -> Data_Out(1B)/1
  Byte_00/1 -> 16_to_1_Byte_Multiplexer/20
  Byte_01/1 -> 16_to_1_Byte_Multiplexer/19
  Byte_02/1 -> 16_to_1_Byte_Multiplexer/18
  Byte_03/1 -> 16_to_1_Byte_Multiplexer/17
  Byte_04/1 -> 16_to_1_Byte_Multiplexer/16
  Byte_05/1 -> 16_to_1_Byte_Multiplexer/15
  Byte_06/1 -> 16_to_1_Byte_Multiplexer/14
  Byte_07/1 -> 16_to_1_Byte_Multiplexer/13
  Byte_08/1 -> 16_to_1_Byte_Multiplexer/12
  Byte_09/1 -> 16_to_1_Byte_Multiplexer/11
  Byte_10/1 -> 16_to_1_Byte_Multiplexer/10
  Byte_11/1 -> 16_to_1_Byte_Multiplexer/9
  Byte_12/1 -> 16_to_1_Byte_Multiplexer/8
  Byte_13/1 -> 16_to_1_Byte_Multiplexer/7
  Byte_14/1 -> 16_to_1_Byte_Multiplexer/6
  Byte_15/1 -> 16_to_1_Byte_Multiplexer/5
  Addr_3(1b)/1 -> 16_to_1_Byte_Multiplexer/1
  Addr_2(1b)/1 -> 16_to_1_Byte_Multiplexer/2
  Addr_1(1b)/1 -> 16_to_1_Byte_Multiplexer/3
  Addr_0(1b)/1 -> 16_to_1_Byte_Multiplexer/4

== system Common_Library/Memory_Blocks/Bit ==
  Select_And_Write(1b) : Inport  OutDataTypeStr=boolean
  Data_In(1b) : Inport  Port=2  OutDataTypeStr=boolean
  CLK : Inport  Port=3  OutDataTypeStr=double
  J-K Flip-Flop : simulink_extras/Flip Flops/J-K Flip-Flop  initial_condition=0
  Logical Operator : Logic  Operator=NOT  IconShape=distinctive  AllPortsSameDT=off  OutDataTypeStr=boolean
  Logical Operator1 : Logic  IconShape=distinctive  AllPortsSameDT=off  OutDataTypeStr=boolean
  Logical Operator2 : Logic  IconShape=distinctive  AllPortsSameDT=off  OutDataTypeStr=boolean
  Terminator : Terminator
  Data_Out(1b) : Outport
  wires:
  Data_In(1b)/1 -> Logical Operator/1, Logical Operator1/2
  J-K Flip-Flop/2 -> Terminator/1
  J-K Flip-Flop/1 -> Data_Out(1b)/1
  CLK/1 -> J-K Flip-Flop/2
  Select_And_Write(1b)/1 -> Logical Operator2/1, Logical Operator1/1
  Logical Operator/1 -> Logical Operator2/2
  Logical Operator1/1 -> J-K Flip-Flop/1
  Logical Operator2/1 -> J-K Flip-Flop/3

== system Common_Library/Memory_Blocks/Byte ==
  Select(1b) : Inport
  Write(1b) : Inport  Port=2
  Data_In(1B) : Inport  Port=3
  CLK : Inport  Port=4  OutDataTypeStr=double
  Bit to Integer Converter : commutil2/Bit to Integer Converter  nbits=8  bitOrder=MSB first  signedOutputValues=Unsigned  outDtype=uint8  outDtypeSigned=Inherit via internal rule
  Bit{0..7} (8 alike) : Common_Library/Memory_Blocks/Bit
  Demux : Demux  Outputs=8
  Integer to Bit Converter : commutil2/Integer to Bit Converter  nbits=8  signedInputValues=Unsigned  bitOrder=MSB first  outDtype=boolean
  Logical Operator : Logic  IconShape=distinctive  AllPortsSameDT=off  OutDataTypeStr=boolean
  Mux : Mux  Inputs=8
  Data_Out(1B) : Outport
  wires:
  Write(1b)/1 -> Logical Operator/2
  Select(1b)/1 -> Logical Operator/1
  Logical Operator/1 -> Bit7/1, Bit6/1, Bit5/1, Bit4/1, Bit3/1, Bit2/1, Bit0/1, Bit1/1
  Data_In(1B)/1 -> Integer to Bit Converter/1
  Demux/7 -> Bit1/2
  Demux/6 -> Bit2/2
  Demux/4 -> Bit4/2
  Demux/3 -> Bit5/2
  Demux/2 -> Bit6/2
  Demux/1 -> Bit7/2
  Demux/8 -> Bit0/2
  Demux/5 -> Bit3/2
  Mux/1 -> Bit to Integer Converter/1
  Bit0/1 -> Mux/8
  Bit1/1 -> Mux/7
  Bit2/1 -> Mux/6
  Bit3/1 -> Mux/5
  Bit4/1 -> Mux/4
  Bit5/1 -> Mux/3
  Bit6/1 -> Mux/2
  Bit7/1 -> Mux/1
  Integer to Bit Converter/1 -> Demux/1
  Bit to Integer Converter/1 -> Data_Out(1B)/1
  CLK/1 -> Bit7/3, Bit6/3, Bit5/3, Bit4/3, Bit3/3, Bit2/3, Bit0/3, Bit1/3

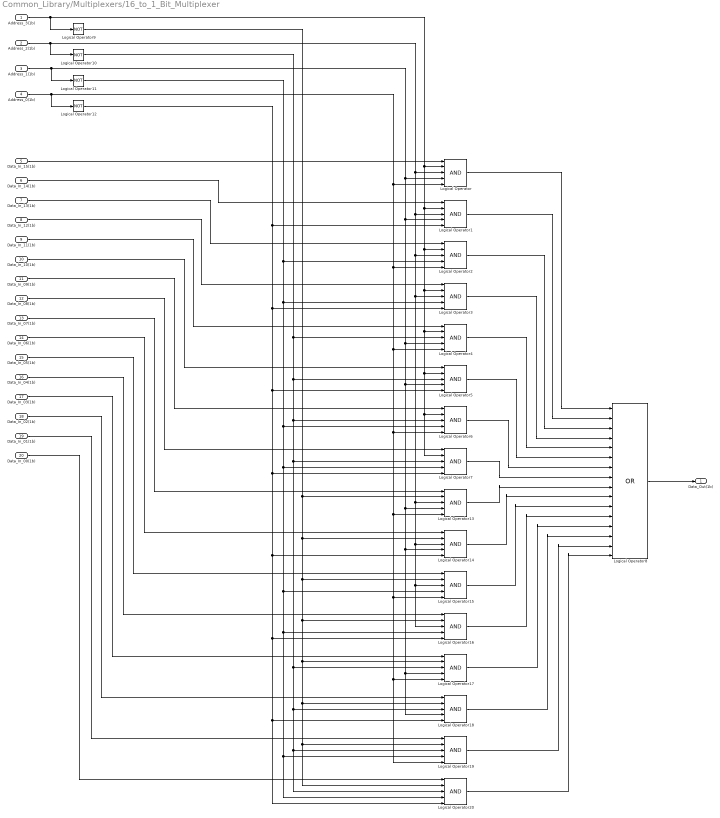
== system Common_Library/Multiplexers/16_to_1_Bit_Multiplexer ==
  Address_3(1b) : Inport
  Address_2(1b) : Inport  Port=2
  Address_1(1b) : Inport  Port=3
  Address_0(1b) : Inport  Port=4
  Data_In_15(1b) : Inport  Port=5
  Data_In_14(1b) : Inport  Port=6
  Data_In_13(1b) : Inport  Port=7
  Data_In_12(1b) : Inport  Port=8
  Data_In_11(1b) : Inport  Port=9
  Data_In_10(1b) : Inport  Port=10
  Data_In_09(1b) : Inport  Port=11
  Data_In_08(1b) : Inport  Port=12
  Data_In_07(1b) : Inport  Port=13
  Data_In_06(1b) : Inport  Port=14
  Data_In_05(1b) : Inport  Port=15
  Data_In_04(1b) : Inport  Port=16
  Data_In_03(1b) : Inport  Port=17
  Data_In_02(1b) : Inport  Port=18
  Data_In_01(1b) : Inport  Port=19
  Data_In_00(1b) : Inport  Port=20
  Logical Operator{,1..7,13..20} (16 alike) : Logic  Inputs=5  IconShape=distinctive  AllPortsSameDT=off  OutDataTypeStr=boolean
  Logical Operator{9..12} (4 alike) : Logic  Operator=NOT  Inputs=4  IconShape=distinctive  AllPortsSameDT=off  OutDataTypeStr=boolean
  Logical Operator8 : Logic  Operator=OR  Inputs=16  IconShape=distinctive  OutDataTypeStr=boolean
  Data_Out(1b) : Outport
  wires:
  Logical Operator12/1 -> Logical Operator7/5, Logical Operator14/5, Logical Operator20/5, Logical Operator18/5, Logical Operator16/5, Logical Operator5/5, Logical Operator3/5, Logical Operator1/5
  Address_0(1b)/1 -> Logical Operator/5, Logical Operator2/5, Logical Operator6/5, Logical Operator13/5, Logical Operator15/5, Logical Operator17/5, Logical Operator19/5, Logical Operator4/5, Logical Operator12/1
  Logical Operator11/1 -> Logical Operator3/4, Logical Operator6/4, Logical Operator7/4, Logical Operator15/4, Logical Operator16/4, Logical Operator19/4, Logical Operator20/4, Logical Operator2/4
  Address_1(1b)/1 -> Logical Operator1/4, Logical Operator4/4, Logical Operator5/4, Logical Operator13/4, Logical Operator14/4, Logical Operator17/4, Logical Operator18/4, Logical Operator/4, Logical Operator11/1
  Logical Operator10/1 -> Logical Operator7/3, Logical Operator17/3, Logical Operator18/3, Logical Operator20/3, Logical Operator19/3, Logical Operator6/3, Logical Operator5/3, Logical Operator4/3
  Address_2(1b)/1 -> Logical Operator3/3, Logical Operator16/3, Logical Operator15/3, Logical Operator14/3, Logical Operator13/3, Logical Operator2/3, Logical Operator1/3, Logical Operator/3, Logical Operator10/1
  Logical Operator9/1 -> Logical Operator13/2, Logical Operator18/2, Logical Operator20/2, Logical Operator19/2, Logical Operator17/2, Logical Operator16/2, Logical Operator15/2, Logical Operator14/2
  Address_3(1b)/1 -> Logical Operator5/2, Logical Operator7/2, Logical Operator6/2, Logical Operator4/2, Logical Operator3/2, Logical Operator2/2, Logical Operator1/2, Logical Operator/2, Logical Operator9/1
  Data_In_00(1b)/1 -> Logical Operator20/1
  Data_In_01(1b)/1 -> Logical Operator19/1
  Data_In_02(1b)/1 -> Logical Operator18/1
  Data_In_03(1b)/1 -> Logical Operator17/1
  Data_In_04(1b)/1 -> Logical Operator16/1
  Data_In_05(1b)/1 -> Logical Operator15/1
  Data_In_06(1b)/1 -> Logical Operator14/1
  Data_In_07(1b)/1 -> Logical Operator13/1
  Logical Operator20/1 -> Logical Operator8/16
  Logical Operator19/1 -> Logical Operator8/15
  Logical Operator18/1 -> Logical Operator8/14
  Logical Operator17/1 -> Logical Operator8/13
  Logical Operator16/1 -> Logical Operator8/12
  Logical Operator15/1 -> Logical Operator8/11
  Logical Operator14/1 -> Logical Operator8/10
  Logical Operator13/1 -> Logical Operator8/9
  Logical Operator8/1 -> Data_Out(1b)/1
  Data_In_15(1b)/1 -> Logical Operator/1
  Data_In_14(1b)/1 -> Logical Operator1/1
  Data_In_13(1b)/1 -> Logical Operator2/1
  Data_In_12(1b)/1 -> Logical Operator3/1
  Data_In_11(1b)/1 -> Logical Operator4/1
  Data_In_10(1b)/1 -> Logical Operator5/1
  Data_In_09(1b)/1 -> Logical Operator6/1
  Data_In_08(1b)/1 -> Logical Operator7/1
  Logical Operator7/1 -> Logical Operator8/8
  Logical Operator6/1 -> Logical Operator8/7
  Logical Operator5/1 -> Logical Operator8/6
  Logical Operator4/1 -> Logical Operator8/5
  Logical Operator3/1 -> Logical Operator8/4
  Logical Operator2/1 -> Logical Operator8/3
  Logical Operator1/1 -> Logical Operator8/2
  Logical Operator/1 -> Logical Operator8/1

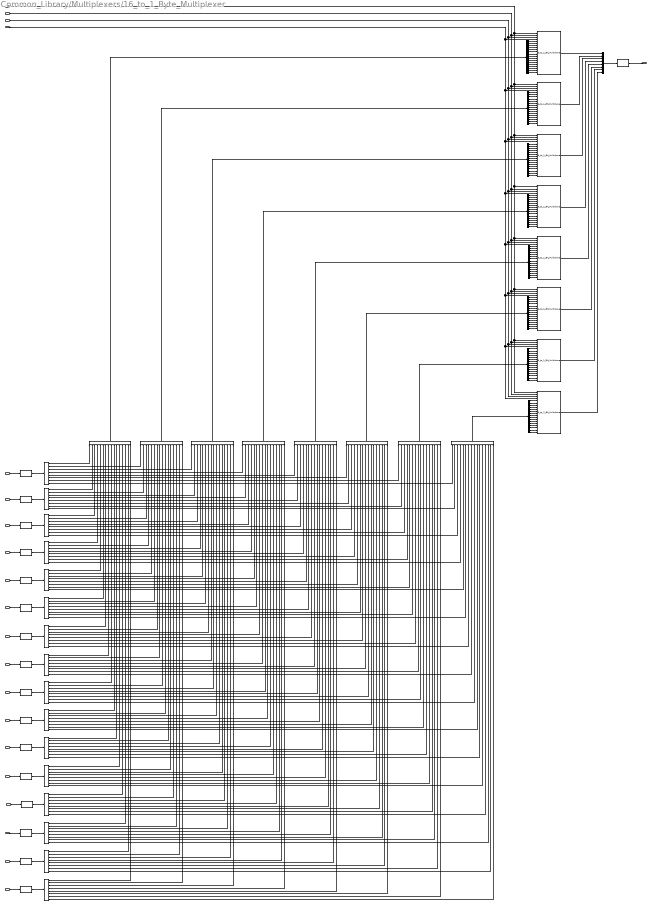
== system Common_Library/Multiplexers/16_to_1_Byte_Multiplexer ==
  Address_3(1b) : Inport
  Address_2(1b) : Inport  Port=2
  Address_1(1b) : Inport  Port=3
  Address_0(1b) : Inport  Port=4
  Data_In_15(1B) : Inport  Port=5
  Data_In_14(1B) : Inport  Port=6
  Data_In_13(1B) : Inport  Port=7
  Data_In_12(1B) : Inport  Port=8
  Data_In_11(1B) : Inport  Port=9
  Data_In_10(1B) : Inport  Port=10
  Data_In_09(1B) : Inport  Port=11
  Data_In_08(1B) : Inport  Port=12
  Data_In_07(1B) : Inport  Port=13
  Data_In_06(1B) : Inport  Port=14
  Data_In_05(1B) : Inport  Port=15
  Data_In_04(1B) : Inport  Port=16
  Data_In_03(1B) : Inport  Port=17
  Data_In_02(1B) : Inport  Port=18
  Data_In_01(1B) : Inport  Port=19
  Data_In_00(1B) : Inport  Port=20
  16_to_1_Bit_Multiplexer(Bit_0) : Common_Library/Multiplexers/16_to_1_Bit_Multiplexer
  16_to_1_Bit_Multiplexer(Bit_1) : Common_Library/Multiplexers/16_to_1_Bit_Multiplexer
  16_to_1_Bit_Multiplexer(Bit_2) : Common_Library/Multiplexers/16_to_1_Bit_Multiplexer
  16_to_1_Bit_Multiplexer(Bit_3) : Common_Library/Multiplexers/16_to_1_Bit_Multiplexer
  16_to_1_Bit_Multiplexer(Bit_4) : Common_Library/Multiplexers/16_to_1_Bit_Multiplexer
  16_to_1_Bit_Multiplexer(Bit_5) : Common_Library/Multiplexers/16_to_1_Bit_Multiplexer
  16_to_1_Bit_Multiplexer(Bit_6) : Common_Library/Multiplexers/16_to_1_Bit_Multiplexer
  16_to_1_Bit_Multiplexer(Bit_7) : Common_Library/Multiplexers/16_to_1_Bit_Multiplexer
  Bit to Integer Converter1 : commutil2/Bit to Integer Converter  nbits=8  bitOrder=MSB first  signedOutputValues=Unsigned  outDtype=uint8  outDtypeSigned=Inherit via internal rule
  Bit_{0..7} (8 alike) : Mux  Inputs=16
  Byte_{0..15} (16 alike) : Demux  Outputs=8
  Demux{,1..7} (8 alike) : Demux  Outputs=16
  Integer to Bit Converter{1..16} (16 alike) : commutil2/Integer to Bit Converter  nbits=8  signedInputValues=Unsigned  bitOrder=MSB first  outDtype=boolean
  Mux : Mux  Inputs=8
  Data_Out(1B) : Outport
  wires:
  Integer to Bit Converter7/1 -> Byte_15/1
  Data_In_15(1B)/1 -> Integer to Bit Converter7/1
  Mux/1 -> Bit to Integer Converter1/1
  Bit to Integer Converter1/1 -> Data_Out(1B)/1
  Bit_0/1 -> Demux7/1
  Bit_1/1 -> Demux6/1
  Bit_2/1 -> Demux5/1
  Bit_3/1 -> Demux4/1
  Bit_4/1 -> Demux3/1
  Bit_5/1 -> Demux2/1
  Bit_6/1 -> Demux1/1
  Bit_7/1 -> Demux/1
  Byte_9/8 -> Bit_0/7
  Byte_7/7 -> Bit_1/9
  Byte_8/1 -> Bit_7/8
  Byte_9/1 -> Bit_7/7
  Byte_10/1 -> Bit_7/6
  Byte_11/1 -> Bit_7/5
  Byte_12/1 -> Bit_7/4
  Byte_13/1 -> Bit_7/3
  Byte_14/1 -> Bit_7/2
  Address_0(1b)/1 -> 16_to_1_Bit_Multiplexer(Bit_5)/4, 16_to_1_Bit_Multiplexer(Bit_0)/4, 16_to_1_Bit_Multiplexer(Bit_1)/4, 16_to_1_Bit_Multiplexer(Bit_2)/4, 16_to_1_Bit_Multiplexer(Bit_3)/4, 16_to_1_Bit_Multiplexer(Bit_4)/4, 16_to_1_Bit_Multiplexer(Bit_6)/4, 16_to_1_Bit_Multiplexer(Bit_7)/4
  Address_1(1b)/1 -> 16_to_1_Bit_Multiplexer(Bit_5)/3, 16_to_1_Bit_Multiplexer(Bit_0)/3, 16_to_1_Bit_Multiplexer(Bit_1)/3, 16_to_1_Bit_Multiplexer(Bit_2)/3, 16_to_1_Bit_Multiplexer(Bit_3)/3, 16_to_1_Bit_Multiplexer(Bit_4)/3, 16_to_1_Bit_Multiplexer(Bit_6)/3, 16_to_1_Bit_Multiplexer(Bit_7)/3
  Address_2(1b)/1 -> 16_to_1_Bit_Multiplexer(Bit_6)/2, 16_to_1_Bit_Multiplexer(Bit_5)/2, 16_to_1_Bit_Multiplexer(Bit_4)/2, 16_to_1_Bit_Multiplexer(Bit_2)/2, 16_to_1_Bit_Multiplexer(Bit_0)/2, 16_to_1_Bit_Multiplexer(Bit_1)/2, 16_to_1_Bit_Multiplexer(Bit_3)/2, 16_to_1_Bit_Multiplexer(Bit_7)/2
  Address_3(1b)/1 -> 16_to_1_Bit_Multiplexer(Bit_5)/1, 16_to_1_Bit_Multiplexer(Bit_0)/1, 16_to_1_Bit_Multiplexer(Bit_1)/1, 16_to_1_Bit_Multiplexer(Bit_2)/1, 16_to_1_Bit_Multiplexer(Bit_3)/1, 16_to_1_Bit_Multiplexer(Bit_4)/1, 16_to_1_Bit_Multiplexer(Bit_6)/1, 16_to_1_Bit_Multiplexer(Bit_7)/1
  16_to_1_Bit_Multiplexer(Bit_4)/1 -> Mux/4
  16_to_1_Bit_Multiplexer(Bit_5)/1 -> Mux/3
  16_to_1_Bit_Multiplexer(Bit_6)/1 -> Mux/2
  16_to_1_Bit_Multiplexer(Bit_7)/1 -> Mux/1
  16_to_1_Bit_Multiplexer(Bit_3)/1 -> Mux/5
  16_to_1_Bit_Multiplexer(Bit_2)/1 -> Mux/6
  16_to_1_Bit_Multiplexer(Bit_1)/1 -> Mux/7
  16_to_1_Bit_Multiplexer(Bit_0)/1 -> Mux/8
  Byte_0/8 -> Bit_0/16
  Byte_1/8 -> Bit_0/15
  Byte_2/8 -> Bit_0/14
  Byte_3/8 -> Bit_0/13
  Byte_4/8 -> Bit_0/12
  Byte_5/8 -> Bit_0/11
  Byte_6/8 -> Bit_0/10
  Byte_7/8 -> Bit_0/9
  Byte_8/8 -> Bit_0/8
  Byte_9/7 -> Bit_1/7
  Byte_10/8 -> Bit_0/6
  Byte_11/8 -> Bit_0/5
  Byte_12/8 -> Bit_0/4
  Byte_13/8 -> Bit_0/3
  Byte_14/8 -> Bit_0/2
  Byte_15/8 -> Bit_0/1
  Byte_0/7 -> Bit_1/16
  Byte_1/7 -> Bit_1/15
  Byte_2/7 -> Bit_1/14
  Byte_3/7 -> Bit_1/13
  Byte_4/7 -> Bit_1/12
  Byte_5/7 -> Bit_1/11
  Byte_6/7 -> Bit_1/10
  Byte_8/7 -> Bit_1/8
  Byte_10/7 -> Bit_1/6
  Byte_11/7 -> Bit_1/5
  Byte_12/7 -> Bit_1/4
  Byte_13/7 -> Bit_1/3
  Byte_14/7 -> Bit_1/2
  Byte_15/7 -> Bit_1/1
  Byte_0/6 -> Bit_2/16
  Byte_1/6 -> Bit_2/15
  Byte_2/6 -> Bit_2/14
  Byte_3/6 -> Bit_2/13
  Byte_4/6 -> Bit_2/12
  Byte_5/6 -> Bit_2/11
  Byte_6/6 -> Bit_2/10
  Byte_7/6 -> Bit_2/9
  Byte_8/6 -> Bit_2/8
  Byte_9/6 -> Bit_2/7
  Byte_10/6 -> Bit_2/6
  Byte_11/6 -> Bit_2/5
  Byte_12/6 -> Bit_2/4
  Byte_13/6 -> Bit_2/3
  Byte_14/6 -> Bit_2/2
  Byte_15/6 -> Bit_2/1
  Byte_0/5 -> Bit_3/16
  Byte_1/5 -> Bit_3/15
  Byte_2/5 -> Bit_3/14
  Byte_3/5 -> Bit_3/13
  Byte_4/5 -> Bit_3/12
  Byte_5/5 -> Bit_3/11
  Byte_6/5 -> Bit_3/10
  Byte_7/5 -> Bit_3/9
  Byte_8/5 -> Bit_3/8
  Byte_9/5 -> Bit_3/7
  Byte_10/5 -> Bit_3/6
  Byte_11/5 -> Bit_3/5
  Byte_12/5 -> Bit_3/4
  Byte_13/5 -> Bit_3/3
  Byte_14/5 -> Bit_3/2
  Byte_15/5 -> Bit_3/1
  Byte_0/4 -> Bit_4/16
  Byte_1/4 -> Bit_4/15
  Byte_2/4 -> Bit_4/14
  Byte_3/4 -> Bit_4/13
  Byte_4/4 -> Bit_4/12
  Byte_5/4 -> Bit_4/11
  Byte_6/4 -> Bit_4/10
  Byte_7/4 -> Bit_4/9
  Byte_8/4 -> Bit_4/8
  Byte_9/4 -> Bit_4/7
  Byte_10/4 -> Bit_4/6
  Byte_11/4 -> Bit_4/5
  Byte_12/4 -> Bit_4/4
  Byte_13/4 -> Bit_4/3
  Byte_14/4 -> Bit_4/2
  Byte_15/4 -> Bit_4/1
  Byte_0/3 -> Bit_5/16
  Byte_1/3 -> Bit_5/15
  Byte_2/3 -> Bit_5/14
  Byte_3/3 -> Bit_5/13
  Byte_4/3 -> Bit_5/12
  Byte_5/3 -> Bit_5/11
  Byte_6/3 -> Bit_5/10
  Byte_7/3 -> Bit_5/9
  Byte_8/3 -> Bit_5/8
  Byte_9/3 -> Bit_5/7
  Byte_10/3 -> Bit_5/6
  Byte_11/3 -> Bit_5/5
  Byte_12/3 -> Bit_5/4
  Byte_13/3 -> Bit_5/3
  Byte_14/3 -> Bit_5/2
  Byte_15/3 -> Bit_5/1
  Byte_0/2 -> Bit_6/16
  Byte_1/2 -> Bit_6/15
  Byte_2/2 -> Bit_6/14
  Byte_3/2 -> Bit_6/13
  Byte_4/2 -> Bit_6/12
  Byte_5/2 -> Bit_6/11
  Byte_6/2 -> Bit_6/10
  Byte_7/2 -> Bit_6/9
  Byte_8/2 -> Bit_6/8
  Byte_9/2 -> Bit_6/7
  Byte_10/2 -> Bit_6/6
  Byte_11/2 -> Bit_6/5
  Byte_12/2 -> Bit_6/4
  Byte_13/2 -> Bit_6/3
  Byte_14/2 -> Bit_6/2
  Byte_15/2 -> Bit_6/1
  Byte_0/1 -> Bit_7/16
  Byte_1/1 -> Bit_7/15
  Byte_2/1 -> Bit_7/14
  Byte_3/1 -> Bit_7/13
  Byte_4/1 -> Bit_7/12
  Byte_5/1 -> Bit_7/11
  Byte_6/1 -> Bit_7/10
  Byte_7/1 -> Bit_7/9
  Byte_15/1 -> Bit_7/1
  Integer to Bit Converter1/1 -> Byte_14/1
  Data_In_14(1B)/1 -> Integer to Bit Converter1/1
  Integer to Bit Converter2/1 -> Byte_13/1
  Data_In_13(1B)/1 -> Integer to Bit Converter2/1
  Integer to Bit Converter3/1 -> Byte_12/1
  Data_In_12(1B)/1 -> Integer to Bit Converter3/1
  Integer to Bit Converter4/1 -> Byte_11/1
  Data_In_11(1B)/1 -> Integer to Bit Converter4/1
  Integer to Bit Converter5/1 -> Byte_10/1
  Data_In_10(1B)/1 -> Integer to Bit Converter5/1
  Integer to Bit Converter6/1 -> Byte_9/1
  Data_In_09(1B)/1 -> Integer to Bit Converter6/1
  Integer to Bit Converter8/1 -> Byte_8/1
  Data_In_08(1B)/1 -> Integer to Bit Converter8/1
  Integer to Bit Converter9/1 -> Byte_7/1
  Data_In_07(1B)/1 -> Integer to Bit Converter9/1
  Integer to Bit Converter10/1 -> Byte_6/1
  Data_In_06(1B)/1 -> Integer to Bit Converter10/1
  Integer to Bit Converter11/1 -> Byte_5/1
  Data_In_05(1B)/1 -> Integer to Bit Converter11/1
  Integer to Bit Converter12/1 -> Byte_4/1
  Data_In_04(1B)/1 -> Integer to Bit Converter12/1
  Integer to Bit Converter13/1 -> Byte_3/1
  Data_In_03(1B)/1 -> Integer to Bit Converter13/1
  Integer to Bit Converter14/1 -> Byte_2/1
  Data_In_02(1B)/1 -> Integer to Bit Converter14/1
  Integer to Bit Converter15/1 -> Byte_1/1
  Data_In_01(1B)/1 -> Integer to Bit Converter15/1
  Integer to Bit Converter16/1 -> Byte_0/1
  Data_In_00(1B)/1 -> Integer to Bit Converter16/1
  Demux/1 -> 16_to_1_Bit_Multiplexer(Bit_7)/5
  Demux/2 -> 16_to_1_Bit_Multiplexer(Bit_7)/6
  Demux/3 -> 16_to_1_Bit_Multiplexer(Bit_7)/7
  Demux/4 -> 16_to_1_Bit_Multiplexer(Bit_7)/8
  Demux/5 -> 16_to_1_Bit_Multiplexer(Bit_7)/9
  Demux/6 -> 16_to_1_Bit_Multiplexer(Bit_7)/10
  Demux/7 -> 16_to_1_Bit_Multiplexer(Bit_7)/11
  Demux/8 -> 16_to_1_Bit_Multiplexer(Bit_7)/12
  Demux/9 -> 16_to_1_Bit_Multiplexer(Bit_7)/13
  Demux/10 -> 16_to_1_Bit_Multiplexer(Bit_7)/14
  Demux/11 -> 16_to_1_Bit_Multiplexer(Bit_7)/15
  Demux/12 -> 16_to_1_Bit_Multiplexer(Bit_7)/16
  Demux/13 -> 16_to_1_Bit_Multiplexer(Bit_7)/17
  Demux/14 -> 16_to_1_Bit_Multiplexer(Bit_7)/18
  Demux/15 -> 16_to_1_Bit_Multiplexer(Bit_7)/19
  Demux/16 -> 16_to_1_Bit_Multiplexer(Bit_7)/20
  Demux1/1 -> 16_to_1_Bit_Multiplexer(Bit_6)/5
  Demux1/2 -> 16_to_1_Bit_Multiplexer(Bit_6)/6
  Demux1/3 -> 16_to_1_Bit_Multiplexer(Bit_6)/7
  Demux1/4 -> 16_to_1_Bit_Multiplexer(Bit_6)/8
  Demux1/5 -> 16_to_1_Bit_Multiplexer(Bit_6)/9
  Demux1/6 -> 16_to_1_Bit_Multiplexer(Bit_6)/10
  Demux1/7 -> 16_to_1_Bit_Multiplexer(Bit_6)/11
  Demux1/8 -> 16_to_1_Bit_Multiplexer(Bit_6)/12
  Demux1/9 -> 16_to_1_Bit_Multiplexer(Bit_6)/13
  Demux1/10 -> 16_to_1_Bit_Multiplexer(Bit_6)/14
  Demux1/11 -> 16_to_1_Bit_Multiplexer(Bit_6)/15
  Demux1/12 -> 16_to_1_Bit_Multiplexer(Bit_6)/16
  Demux1/13 -> 16_to_1_Bit_Multiplexer(Bit_6)/17
  Demux1/14 -> 16_to_1_Bit_Multiplexer(Bit_6)/18
  Demux1/15 -> 16_to_1_Bit_Multiplexer(Bit_6)/19
  Demux1/16 -> 16_to_1_Bit_Multiplexer(Bit_6)/20
  Demux2/1 -> 16_to_1_Bit_Multiplexer(Bit_5)/5
  Demux2/2 -> 16_to_1_Bit_Multiplexer(Bit_5)/6
  Demux2/3 -> 16_to_1_Bit_Multiplexer(Bit_5)/7
  Demux2/4 -> 16_to_1_Bit_Multiplexer(Bit_5)/8
  Demux2/5 -> 16_to_1_Bit_Multiplexer(Bit_5)/9
  Demux2/6 -> 16_to_1_Bit_Multiplexer(Bit_5)/10
  Demux2/7 -> 16_to_1_Bit_Multiplexer(Bit_5)/11
  Demux2/8 -> 16_to_1_Bit_Multiplexer(Bit_5)/12
  Demux2/9 -> 16_to_1_Bit_Multiplexer(Bit_5)/13
  Demux2/10 -> 16_to_1_Bit_Multiplexer(Bit_5)/14
  Demux2/11 -> 16_to_1_Bit_Multiplexer(Bit_5)/15
  Demux2/12 -> 16_to_1_Bit_Multiplexer(Bit_5)/16
  Demux2/13 -> 16_to_1_Bit_Multiplexer(Bit_5)/17
  Demux2/14 -> 16_to_1_Bit_Multiplexer(Bit_5)/18
  Demux2/15 -> 16_to_1_Bit_Multiplexer(Bit_5)/19
  Demux2/16 -> 16_to_1_Bit_Multiplexer(Bit_5)/20
  Demux3/1 -> 16_to_1_Bit_Multiplexer(Bit_4)/5
  Demux3/2 -> 16_to_1_Bit_Multiplexer(Bit_4)/6
  Demux3/3 -> 16_to_1_Bit_Multiplexer(Bit_4)/7
  Demux3/4 -> 16_to_1_Bit_Multiplexer(Bit_4)/8
  Demux3/5 -> 16_to_1_Bit_Multiplexer(Bit_4)/9
  Demux3/6 -> 16_to_1_Bit_Multiplexer(Bit_4)/10
  Demux3/7 -> 16_to_1_Bit_Multiplexer(Bit_4)/11
  Demux3/8 -> 16_to_1_Bit_Multiplexer(Bit_4)/12
  Demux3/9 -> 16_to_1_Bit_Multiplexer(Bit_4)/13
  Demux3/10 -> 16_to_1_Bit_Multiplexer(Bit_4)/14
  Demux3/11 -> 16_to_1_Bit_Multiplexer(Bit_4)/15
  Demux3/12 -> 16_to_1_Bit_Multiplexer(Bit_4)/16
  Demux3/13 -> 16_to_1_Bit_Multiplexer(Bit_4)/17
  Demux3/14 -> 16_to_1_Bit_Multiplexer(Bit_4)/18
  Demux3/15 -> 16_to_1_Bit_Multiplexer(Bit_4)/19
  Demux3/16 -> 16_to_1_Bit_Multiplexer(Bit_4)/20
  Demux4/1 -> 16_to_1_Bit_Multiplexer(Bit_3)/5
  Demux4/2 -> 16_to_1_Bit_Multiplexer(Bit_3)/6
  Demux4/3 -> 16_to_1_Bit_Multiplexer(Bit_3)/7
  Demux4/4 -> 16_to_1_Bit_Multiplexer(Bit_3)/8
  Demux4/5 -> 16_to_1_Bit_Multiplexer(Bit_3)/9
  Demux4/6 -> 16_to_1_Bit_Multiplexer(Bit_3)/10
  Demux4/7 -> 16_to_1_Bit_Multiplexer(Bit_3)/11
  Demux4/8 -> 16_to_1_Bit_Multiplexer(Bit_3)/12
  Demux4/9 -> 16_to_1_Bit_Multiplexer(Bit_3)/13
  Demux4/10 -> 16_to_1_Bit_Multiplexer(Bit_3)/14
  Demux4/11 -> 16_to_1_Bit_Multiplexer(Bit_3)/15
  Demux4/12 -> 16_to_1_Bit_Multiplexer(Bit_3)/16
  Demux4/13 -> 16_to_1_Bit_Multiplexer(Bit_3)/17
  Demux4/14 -> 16_to_1_Bit_Multiplexer(Bit_3)/18
  Demux4/15 -> 16_to_1_Bit_Multiplexer(Bit_3)/19
  Demux4/16 -> 16_to_1_Bit_Multiplexer(Bit_3)/20
  Demux5/1 -> 16_to_1_Bit_Multiplexer(Bit_2)/5
  Demux5/2 -> 16_to_1_Bit_Multiplexer(Bit_2)/6
  Demux5/3 -> 16_to_1_Bit_Multiplexer(Bit_2)/7
  Demux5/4 -> 16_to_1_Bit_Multiplexer(Bit_2)/8
  Demux5/5 -> 16_to_1_Bit_Multiplexer(Bit_2)/9
  Demux5/6 -> 16_to_1_Bit_Multiplexer(Bit_2)/10
  Demux5/7 -> 16_to_1_Bit_Multiplexer(Bit_2)/11
  Demux5/8 -> 16_to_1_Bit_Multiplexer(Bit_2)/12
  Demux5/9 -> 16_to_1_Bit_Multiplexer(Bit_2)/13
  Demux5/10 -> 16_to_1_Bit_Multiplexer(Bit_2)/14
  Demux5/11 -> 16_to_1_Bit_Multiplexer(Bit_2)/15
  Demux5/12 -> 16_to_1_Bit_Multiplexer(Bit_2)/16
  Demux5/13 -> 16_to_1_Bit_Multiplexer(Bit_2)/17
  Demux5/14 -> 16_to_1_Bit_Multiplexer(Bit_2)/18
  Demux5/15 -> 16_to_1_Bit_Multiplexer(Bit_2)/19
  Demux5/16 -> 16_to_1_Bit_Multiplexer(Bit_2)/20
  Demux6/1 -> 16_to_1_Bit_Multiplexer(Bit_1)/5
  Demux6/2 -> 16_to_1_Bit_Multiplexer(Bit_1)/6
  Demux6/3 -> 16_to_1_Bit_Multiplexer(Bit_1)/7
  Demux6/4 -> 16_to_1_Bit_Multiplexer(Bit_1)/8
  Demux6/5 -> 16_to_1_Bit_Multiplexer(Bit_1)/9
  Demux6/6 -> 16_to_1_Bit_Multiplexer(Bit_1)/10
  Demux6/7 -> 16_to_1_Bit_Multiplexer(Bit_1)/11
  Demux6/8 -> 16_to_1_Bit_Multiplexer(Bit_1)/12
  Demux6/9 -> 16_to_1_Bit_Multiplexer(Bit_1)/13
  Demux6/10 -> 16_to_1_Bit_Multiplexer(Bit_1)/14
  Demux6/11 -> 16_to_1_Bit_Multiplexer(Bit_1)/15
  Demux6/12 -> 16_to_1_Bit_Multiplexer(Bit_1)/16
  Demux6/13 -> 16_to_1_Bit_Multiplexer(Bit_1)/17
  Demux6/14 -> 16_to_1_Bit_Multiplexer(Bit_1)/18
  Demux6/15 -> 16_to_1_Bit_Multiplexer(Bit_1)/19
  Demux6/16 -> 16_to_1_Bit_Multiplexer(Bit_1)/20
  Demux7/1 -> 16_to_1_Bit_Multiplexer(Bit_0)/5
  Demux7/2 -> 16_to_1_Bit_Multiplexer(Bit_0)/6
  Demux7/3 -> 16_to_1_Bit_Multiplexer(Bit_0)/7
  Demux7/4 -> 16_to_1_Bit_Multiplexer(Bit_0)/8
  Demux7/5 -> 16_to_1_Bit_Multiplexer(Bit_0)/9
  Demux7/6 -> 16_to_1_Bit_Multiplexer(Bit_0)/10
  Demux7/7 -> 16_to_1_Bit_Multiplexer(Bit_0)/11
  Demux7/8 -> 16_to_1_Bit_Multiplexer(Bit_0)/12
  Demux7/9 -> 16_to_1_Bit_Multiplexer(Bit_0)/13
  Demux7/10 -> 16_to_1_Bit_Multiplexer(Bit_0)/14
  Demux7/11 -> 16_to_1_Bit_Multiplexer(Bit_0)/15
  Demux7/12 -> 16_to_1_Bit_Multiplexer(Bit_0)/16
  Demux7/13 -> 16_to_1_Bit_Multiplexer(Bit_0)/17
  Demux7/14 -> 16_to_1_Bit_Multiplexer(Bit_0)/18
  Demux7/15 -> 16_to_1_Bit_Multiplexer(Bit_0)/19
  Demux7/16 -> 16_to_1_Bit_Multiplexer(Bit_0)/20
